simulink model "Sim_2"  (R2022b)
settings: Solver=ode4  StartTime=0.0  StopTime=10  FixedStep=0.001  RelTol=1e-3  EnableMultiTasking=on
settings Model: Creator=J  LastModifiedBy=J
settings DataIOCC: SaveFormat=Array  SignalLoggingSaveFormat=ModelDataLogs  ReturnWorkspaceOutputs=off  SignalLoggingName=sigsOut
settings OptimizationCC: BooleanDataType=off
settings DebuggingCC: SaveWithParameterizedLinksMsg=none  UnderspecifiedInitializationDetection=Classic  MergeDetectMultiDrivingBlocksExec=none  SignalResolutionControl=TryResolveAllWithWarning  MultiTaskDSMMsg=warning  MultiTaskCondExecSysMsg=none  UnconnectedInputMsg=warning  UnconnectedOutputMsg=warning  UnconnectedLineMsg=warning
settings HardwareCC: ProdBitPerPointer=32  ProdBitPerSizeT=32  ProdBitPerPtrDiffT=32  ProdLargestAtomicFloat=None  ProdIntDivRoundTo=Undefined  ProdEndianess=Unspecified  ProdWordSize=32  ProdHWDeviceType=32-bit Generic  TargetUnknown=on
settings ModelReferenceCC: PropagateSignalLabelsOutOfModel=off
settings GRTTargetCC: CombineOutputUpdateFcns=off  GRTInterface=on
settings ConfigComp: CovMetricSettings=dw  CovSaveCumulativeToWorkspaceVar=on  CovSaveSingleToWorkspaceVar=on

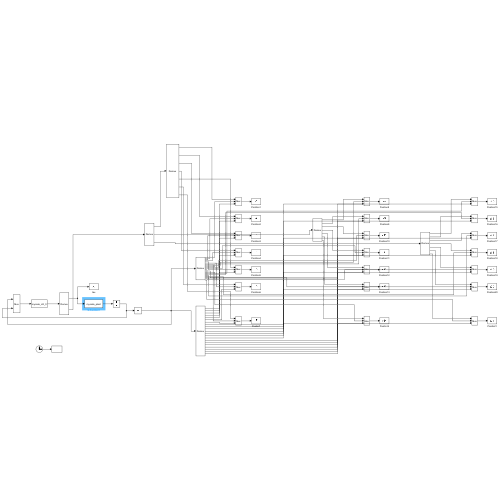
[thumbnail: Simulink's stored preview of the top-level diagram]
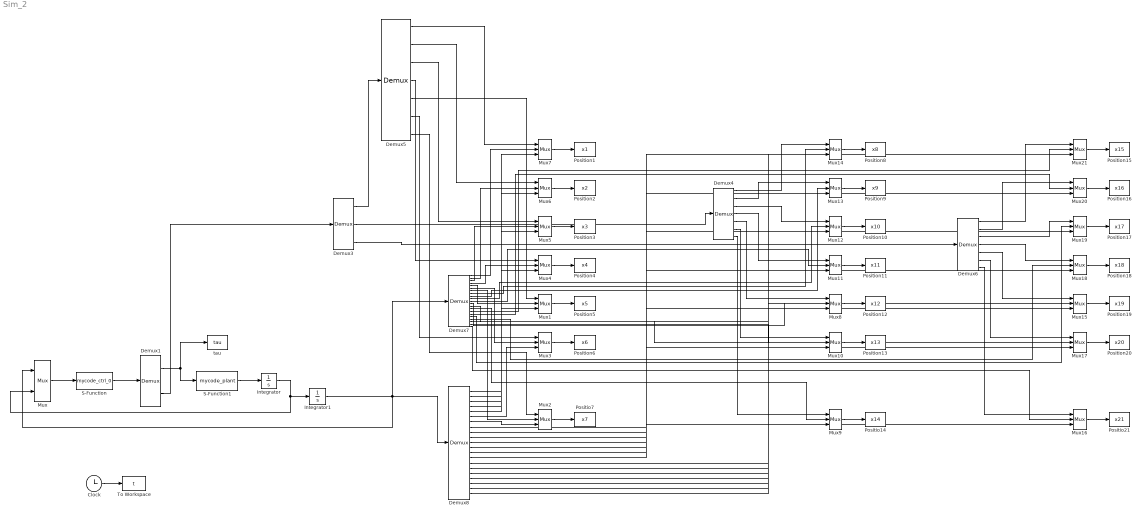
== system Sim_2 ==
  " Position9" : ToWorkspace  VariableName=x9  SampleTime=-1
  Clock : Clock
  Demux1 : Demux  Outputs=2
      settings: DisplayOption=none
  Demux3 : Demux  Outputs=3
      settings: DisplayOption=none
  Demux4 : Demux  Outputs=7
      settings: DisplayOption=none
  Demux5 : Demux  Outputs=7
      settings: DisplayOption=none
  Demux6 : Demux  Outputs=7
      settings: DisplayOption=none
  Demux7 : Demux  Outputs=21
      settings: DisplayOption=none
  Demux8 : Demux  Outputs=21
      settings: DisplayOption=none
  Integrator : Integrator
  Integrator1 : Integrator
  Mux : Mux  Inputs=2
  Mux{1..21} (21 alike) : Mux  Inputs=3
  Positio14 : ToWorkspace  VariableName=x14  SampleTime=-1
  Positio21 : ToWorkspace  VariableName=x21  SampleTime=-1
  Positio7 : ToWorkspace  VariableName=x7  SampleTime=-1
  Position1 : ToWorkspace  VariableName=x1  SampleTime=-1
  Position10 : ToWorkspace  VariableName=x10  SampleTime=-1
  Position11 : ToWorkspace  VariableName=x11  SampleTime=-1
  Position12 : ToWorkspace  VariableName=x12  SampleTime=-1
  Position13 : ToWorkspace  VariableName=x13  SampleTime=-1
  Position15 : ToWorkspace  VariableName=x15  SampleTime=-1
  Position16 : ToWorkspace  VariableName=x16  SampleTime=-1
  Position17 : ToWorkspace  VariableName=x17  SampleTime=-1
  Position18 : ToWorkspace  VariableName=x18  SampleTime=-1
  Position19 : ToWorkspace  VariableName=x19  SampleTime=-1
  Position2 : ToWorkspace  VariableName=x2  SampleTime=-1
  Position20 : ToWorkspace  VariableName=x20  SampleTime=-1
  Position3 : ToWorkspace  VariableName=x3  SampleTime=-1
  Position4 : ToWorkspace  VariableName=x4  SampleTime=-1
  Position5 : ToWorkspace  VariableName=x5  SampleTime=-1
  Position6 : ToWorkspace  VariableName=x6  SampleTime=-1
  Position8 : ToWorkspace  VariableName=x8  SampleTime=-1
  S-Function : S-Function  FunctionName=mycode_ctrl_0  SFunctionDeploymentMode=off  EnableBusSupport=off
  S-Function1 : S-Function  FunctionName=mycode_plant  SFunctionDeploymentMode=off  EnableBusSupport=off
  To Workspace : ToWorkspace  VariableName=t  SampleTime=-1
  tau : ToWorkspace  VariableName=tau  SampleTime=-1
  wires:
  Mux/1 -> S-Function/1
  Mux2/1 -> Positio7/1
  Mux3/1 -> Position6/1
  Clock/1 -> To Workspace/1
  Mux1/1 -> Position5/1
  Mux4/1 -> Position4/1
  Mux5/1 -> Position3/1
  Mux6/1 -> Position2/1
  Mux7/1 -> Position1/1
  S-Function/1 -> Demux1/1
  Demux1/1 -> tau/1, S-Function1/1
  Demux1/2 -> Demux3/1
  Mux8/1 -> Position12/1
  Mux12/1 -> Position10/1
  Mux14/1 -> Position8/1
  Mux9/1 -> Positio14/1
  Mux10/1 -> Position13/1
  Mux13/1 -> " Position9"/1
  Mux11/1 -> Position11/1
  Mux15/1 -> Position19/1
  Mux19/1 -> Position17/1
  Mux21/1 -> Position15/1
  Mux16/1 -> Positio21/1
  Mux17/1 -> Position20/1
  Mux20/1 -> Position16/1
  Mux18/1 -> Position18/1
  Demux3/1 -> Demux5/1
  Demux3/2 -> Demux4/1
  Demux3/3 -> Demux6/1
  Demux4/1 -> Mux14/1
  Demux4/2 -> Mux13/1
  Demux4/3 -> Mux12/1
  Demux4/4 -> Mux11/1
  Demux4/5 -> Mux8/1
  Demux4/6 -> Mux10/1
  Demux4/7 -> Mux9/1
  Demux6/1 -> Mux21/1
  Demux6/2 -> Mux20/1
  Demux6/3 -> Mux19/1
  Demux6/4 -> Mux18/1
  Demux6/5 -> Mux15/1
  Demux6/6 -> Mux17/1
  Demux6/7 -> Mux16/1
  Integrator/1 -> Mux/2, Integrator1/1
  Integrator1/1 -> Demux7/1, Demux8/1, Mux/1
  Demux5/1 -> Mux7/1
  Demux5/2 -> Mux6/1
  Demux5/3 -> Mux5/1
  Demux5/4 -> Mux4/1
  Demux5/5 -> Mux1/1
  Demux5/6 -> Mux3/1
  Demux5/7 -> Mux2/1
  Demux7/1 -> Mux7/2
  Demux7/2 -> Mux6/2
  Demux7/3 -> Mux5/2
  Demux7/4 -> Mux4/2
  Demux7/5 -> Mux1/2
  Demux7/6 -> Mux3/2
  Demux7/7 -> Mux2/2
  Demux7/8 -> Mux14/2
  Demux7/9 -> Mux13/2
  Demux7/10 -> Mux12/2
  Demux7/11 -> Mux11/2
  Demux7/12 -> Mux8/2
  Demux7/13 -> Mux10/2
  Demux7/14 -> Mux9/2
  Demux7/15 -> Mux21/2
  Demux7/16 -> Mux20/2
  Demux7/17 -> Mux19/2
  Demux7/18 -> Mux18/2
  Demux7/19 -> Mux15/2
  Demux7/20 -> Mux17/2
  Demux7/21 -> Mux16/2
  Demux8/1 -> Mux7/3
  Demux8/2 -> Mux6/3
  Demux8/3 -> Mux5/3
  Demux8/4 -> Mux4/3
  Demux8/5 -> Mux1/3
  Demux8/6 -> Mux3/3
  Demux8/7 -> Mux2/3
  Demux8/8 -> Mux14/3
  Demux8/9 -> Mux13/3
  Demux8/10 -> Mux12/3
  Demux8/11 -> Mux11/3
  Demux8/12 -> Mux8/3
  Demux8/13 -> Mux10/3
  Demux8/14 -> Mux9/3
  Demux8/15 -> Mux21/3
  Demux8/16 -> Mux20/3
  Demux8/17 -> Mux19/3
  Demux8/18 -> Mux18/3
  Demux8/19 -> Mux15/3
  Demux8/20 -> Mux17/3
  Demux8/21 -> Mux16/3
  S-Function1/1 -> Integrator/1
